simulink model "Teste"  (R2020b)
settings: Solver=VariableStepAuto  StartTime=0.0  StopTime=10.0  RelTol=1e-3
undefined symbols (not defined in the file or in its folder): des, SELECT, T
libraries: simulink x8
(part 3 of 3)

== system Teste/Router5/Clocked FIFO1 ==
  Event-Based Random Number : EventBasedRandomNumber  Distribution=Gaussian (normal)  meanNorm=E  stdNorm=S
  FIFO Queue : FIFOQueue  Capacity=F  StatNumberInBlock=on
      settings: OutputPortMap=o1
  Release Gate : ReleaseGate  OpenGateUpon=Function call from port fcn
  Time-Based Function-Call Generator : TimeBasedFunctionCallGenerator  EventGenerationMode=Period from port  Period=T
  Input : PMIOPort  Side=Left
  Output : PMIOPort  Port=2  Side=Right
  #n : Outport
  wires:
  Event-Based Random Number/1 -> Time-Based Function-Call Generator/1
  FIFO Queue/1 -> #n/1
  Time-Based Function-Call Generator/1 -> Release Gate/1
  connections:
  FIFO Queue/RConn1 -- Release Gate/LConn1
  Release Gate/RConn1 -- Output/RConn1
  FIFO Queue/LConn1 -- Input/RConn1

== system Teste/Router5/Clocked FIFO2 ==
  Event-Based Random Number : EventBasedRandomNumber  Distribution=Gaussian (normal)  meanNorm=E  stdNorm=S
  FIFO Queue : FIFOQueue  Capacity=F  StatNumberInBlock=on
      settings: OutputPortMap=o1
  Release Gate : ReleaseGate  OpenGateUpon=Function call from port fcn
  Time-Based Function-Call Generator : TimeBasedFunctionCallGenerator  EventGenerationMode=Period from port  Period=T
  Input : PMIOPort  Side=Left
  Output : PMIOPort  Port=2  Side=Right
  #n : Outport
  wires:
  Event-Based Random Number/1 -> Time-Based Function-Call Generator/1
  FIFO Queue/1 -> #n/1
  Time-Based Function-Call Generator/1 -> Release Gate/1
  connections:
  FIFO Queue/RConn1 -- Release Gate/LConn1
  Release Gate/RConn1 -- Output/RConn1
  FIFO Queue/LConn1 -- Input/RConn1

== system Teste/Router5/Clocked FIFO3 ==
  Event-Based Random Number : EventBasedRandomNumber  Distribution=Gaussian (normal)  meanNorm=E  stdNorm=S
  FIFO Queue : FIFOQueue  Capacity=F  StatNumberInBlock=on
      settings: OutputPortMap=o1
  Release Gate : ReleaseGate  OpenGateUpon=Function call from port fcn
  Time-Based Function-Call Generator : TimeBasedFunctionCallGenerator  EventGenerationMode=Period from port  Period=T
  Input : PMIOPort  Side=Left
  Output : PMIOPort  Port=2  Side=Right
  #n : Outport
  wires:
  Event-Based Random Number/1 -> Time-Based Function-Call Generator/1
  FIFO Queue/1 -> #n/1
  Time-Based Function-Call Generator/1 -> Release Gate/1
  connections:
  FIFO Queue/RConn1 -- Release Gate/LConn1
  Release Gate/RConn1 -- Output/RConn1
  FIFO Queue/LConn1 -- Input/RConn1

== system Teste/Router5/Clocked FIFO4 ==
  Event-Based Random Number : EventBasedRandomNumber  Distribution=Gaussian (normal)  meanNorm=E  stdNorm=S
  FIFO Queue : FIFOQueue  Capacity=F  StatNumberInBlock=on
      settings: OutputPortMap=o1
  Release Gate : ReleaseGate  OpenGateUpon=Function call from port fcn
  Time-Based Function-Call Generator : TimeBasedFunctionCallGenerator  EventGenerationMode=Period from port  Period=T
  Input : PMIOPort  Side=Left
  Output : PMIOPort  Port=2  Side=Right
  #n : Outport
  wires:
  Event-Based Random Number/1 -> Time-Based Function-Call Generator/1
  FIFO Queue/1 -> #n/1
  Time-Based Function-Call Generator/1 -> Release Gate/1
  connections:
  FIFO Queue/RConn1 -- Release Gate/LConn1
  Release Gate/RConn1 -- Output/RConn1
  FIFO Queue/LConn1 -- Input/RConn1

== system Teste/Router5/Clocked FIFO5 ==
  Event-Based Random Number : EventBasedRandomNumber  Distribution=Gaussian (normal)  meanNorm=E  stdNorm=S
  FIFO Queue : FIFOQueue  Capacity=F  StatNumberInBlock=on
      settings: OutputPortMap=o1
  Release Gate : ReleaseGate  OpenGateUpon=Function call from port fcn
  Time-Based Function-Call Generator : TimeBasedFunctionCallGenerator  EventGenerationMode=Period from port  Period=T
  Input : PMIOPort  Side=Left
  Output : PMIOPort  Port=2  Side=Right
  #n : Outport
  wires:
  Event-Based Random Number/1 -> Time-Based Function-Call Generator/1
  FIFO Queue/1 -> #n/1
  Time-Based Function-Call Generator/1 -> Release Gate/1
  connections:
  FIFO Queue/RConn1 -- Release Gate/LConn1
  Release Gate/RConn1 -- Output/RConn1
  FIFO Queue/LConn1 -- Input/RConn1

== system Teste/Router6/Attribute Function ==
  MATLAB Function : MATLAB Function  TreatAsAtomicUnit=on
  __DMLF__EDE2FCE__ : EntityDepartureFunctionCallGenerator  TimingFunctionCallF1=Before entity departure  IsInsideAFB=on
  __DMLF__GA__ : GetAttribute  AttributeName=DST|ME  AttributeMissing=Error|Error  AttributeDefaultValue=1|1  AttributeTreatAsVector=1|1  AttributeSendTiming=Before entity departure|Before entity departure  EvaluatedDefaultAttributeValue={ [];[]}  IsInsideAFB=on
      settings: OutputPortMap=o1,o2
  __DMLF__SA__ : SetAttribute  AttributeName=RT  AttributeFrom=Signal port  EvaluatedAttributeValue={ []}  IsInsideAFB=on
  IN : PMIOPort  Side=Left
  OUT : PMIOPort  Port=2  Side=Right
  wires:
  MATLAB Function/1(out_RT) -> __DMLF__SA__/1
  __DMLF__GA__/2 -> MATLAB Function/2(ME)
  __DMLF__GA__/1 -> MATLAB Function/1(DST)
  __DMLF__EDE2FCE__/1 -> MATLAB Function/Trigger
  connections:
  __DMLF__SA__/RConn1 -- OUT/RConn1
  IN/RConn1 -- __DMLF__GA__/LConn1
  __DMLF__GA__/RConn1 -- __DMLF__EDE2FCE__/LConn1
  __DMLF__SA__/LConn1 -- __DMLF__EDE2FCE__/RConn1

== system Teste/Router6/Clocked FIFO1 ==
  Event-Based Random Number : EventBasedRandomNumber  Distribution=Gaussian (normal)  meanNorm=E  stdNorm=S
  FIFO Queue : FIFOQueue  Capacity=F  StatNumberInBlock=on
      settings: OutputPortMap=o1
  Release Gate : ReleaseGate  OpenGateUpon=Function call from port fcn
  Time-Based Function-Call Generator : TimeBasedFunctionCallGenerator  EventGenerationMode=Period from port  Period=T
  Input : PMIOPort  Side=Left
  Output : PMIOPort  Port=2  Side=Right
  #n : Outport
  wires:
  Event-Based Random Number/1 -> Time-Based Function-Call Generator/1
  FIFO Queue/1 -> #n/1
  Time-Based Function-Call Generator/1 -> Release Gate/1
  connections:
  FIFO Queue/RConn1 -- Release Gate/LConn1
  Release Gate/RConn1 -- Output/RConn1
  FIFO Queue/LConn1 -- Input/RConn1

== system Teste/Router6/Clocked FIFO2 ==
  Event-Based Random Number : EventBasedRandomNumber  Distribution=Gaussian (normal)  meanNorm=E  stdNorm=S
  FIFO Queue : FIFOQueue  Capacity=F  StatNumberInBlock=on
      settings: OutputPortMap=o1
  Release Gate : ReleaseGate  OpenGateUpon=Function call from port fcn
  Time-Based Function-Call Generator : TimeBasedFunctionCallGenerator  EventGenerationMode=Period from port  Period=T
  Input : PMIOPort  Side=Left
  Output : PMIOPort  Port=2  Side=Right
  #n : Outport
  wires:
  Event-Based Random Number/1 -> Time-Based Function-Call Generator/1
  FIFO Queue/1 -> #n/1
  Time-Based Function-Call Generator/1 -> Release Gate/1
  connections:
  FIFO Queue/RConn1 -- Release Gate/LConn1
  Release Gate/RConn1 -- Output/RConn1
  FIFO Queue/LConn1 -- Input/RConn1

== system Teste/Router6/Clocked FIFO3 ==
  Event-Based Random Number : EventBasedRandomNumber  Distribution=Gaussian (normal)  meanNorm=E  stdNorm=S
  FIFO Queue : FIFOQueue  Capacity=F  StatNumberInBlock=on
      settings: OutputPortMap=o1
  Release Gate : ReleaseGate  OpenGateUpon=Function call from port fcn
  Time-Based Function-Call Generator : TimeBasedFunctionCallGenerator  EventGenerationMode=Period from port  Period=T
  Input : PMIOPort  Side=Left
  Output : PMIOPort  Port=2  Side=Right
  #n : Outport
  wires:
  Event-Based Random Number/1 -> Time-Based Function-Call Generator/1
  FIFO Queue/1 -> #n/1
  Time-Based Function-Call Generator/1 -> Release Gate/1
  connections:
  FIFO Queue/RConn1 -- Release Gate/LConn1
  Release Gate/RConn1 -- Output/RConn1
  FIFO Queue/LConn1 -- Input/RConn1

== system Teste/Router6/Clocked FIFO4 ==
  Event-Based Random Number : EventBasedRandomNumber  Distribution=Gaussian (normal)  meanNorm=E  stdNorm=S
  FIFO Queue : FIFOQueue  Capacity=F  StatNumberInBlock=on
      settings: OutputPortMap=o1
  Release Gate : ReleaseGate  OpenGateUpon=Function call from port fcn
  Time-Based Function-Call Generator : TimeBasedFunctionCallGenerator  EventGenerationMode=Period from port  Period=T
  Input : PMIOPort  Side=Left
  Output : PMIOPort  Port=2  Side=Right
  #n : Outport
  wires:
  Event-Based Random Number/1 -> Time-Based Function-Call Generator/1
  FIFO Queue/1 -> #n/1
  Time-Based Function-Call Generator/1 -> Release Gate/1
  connections:
  FIFO Queue/RConn1 -- Release Gate/LConn1
  Release Gate/RConn1 -- Output/RConn1
  FIFO Queue/LConn1 -- Input/RConn1

== system Teste/Router6/Clocked FIFO5 ==
  Event-Based Random Number : EventBasedRandomNumber  Distribution=Gaussian (normal)  meanNorm=E  stdNorm=S
  FIFO Queue : FIFOQueue  Capacity=F  StatNumberInBlock=on
      settings: OutputPortMap=o1
  Release Gate : ReleaseGate  OpenGateUpon=Function call from port fcn
  Time-Based Function-Call Generator : TimeBasedFunctionCallGenerator  EventGenerationMode=Period from port  Period=T
  Input : PMIOPort  Side=Left
  Output : PMIOPort  Port=2  Side=Right
  #n : Outport
  wires:
  Event-Based Random Number/1 -> Time-Based Function-Call Generator/1
  FIFO Queue/1 -> #n/1
  Time-Based Function-Call Generator/1 -> Release Gate/1
  connections:
  FIFO Queue/RConn1 -- Release Gate/LConn1
  Release Gate/RConn1 -- Output/RConn1
  FIFO Queue/LConn1 -- Input/RConn1

== system Teste/Router7/Attribute Function ==
  MATLAB Function : MATLAB Function  TreatAsAtomicUnit=on
  __DMLF__EDE2FCE__ : EntityDepartureFunctionCallGenerator  TimingFunctionCallF1=Before entity departure  IsInsideAFB=on
  __DMLF__GA__ : GetAttribute  AttributeName=DST|ME  AttributeMissing=Error|Error  AttributeDefaultValue=1|1  AttributeTreatAsVector=1|1  AttributeSendTiming=Before entity departure|Before entity departure  EvaluatedDefaultAttributeValue={ [];[]}  IsInsideAFB=on
      settings: OutputPortMap=o1,o2
  __DMLF__SA__ : SetAttribute  AttributeName=RT  AttributeFrom=Signal port  EvaluatedAttributeValue={ []}  IsInsideAFB=on
  IN : PMIOPort  Side=Left
  OUT : PMIOPort  Port=2  Side=Right
  wires:
  MATLAB Function/1(out_RT) -> __DMLF__SA__/1
  __DMLF__GA__/2 -> MATLAB Function/2(ME)
  __DMLF__GA__/1 -> MATLAB Function/1(DST)
  __DMLF__EDE2FCE__/1 -> MATLAB Function/Trigger
  connections:
  __DMLF__SA__/RConn1 -- OUT/RConn1
  IN/RConn1 -- __DMLF__GA__/LConn1
  __DMLF__GA__/RConn1 -- __DMLF__EDE2FCE__/LConn1
  __DMLF__SA__/LConn1 -- __DMLF__EDE2FCE__/RConn1

== system Teste/Router7/Clocked FIFO1 ==
  Event-Based Random Number : EventBasedRandomNumber  Distribution=Gaussian (normal)  meanNorm=E  stdNorm=S
  FIFO Queue : FIFOQueue  Capacity=F  StatNumberInBlock=on
      settings: OutputPortMap=o1
  Release Gate : ReleaseGate  OpenGateUpon=Function call from port fcn
  Time-Based Function-Call Generator : TimeBasedFunctionCallGenerator  EventGenerationMode=Period from port  Period=T
  Input : PMIOPort  Side=Left
  Output : PMIOPort  Port=2  Side=Right
  #n : Outport
  wires:
  Event-Based Random Number/1 -> Time-Based Function-Call Generator/1
  FIFO Queue/1 -> #n/1
  Time-Based Function-Call Generator/1 -> Release Gate/1
  connections:
  FIFO Queue/RConn1 -- Release Gate/LConn1
  Release Gate/RConn1 -- Output/RConn1
  FIFO Queue/LConn1 -- Input/RConn1

== system Teste/Router7/Clocked FIFO2 ==
  Event-Based Random Number : EventBasedRandomNumber  Distribution=Gaussian (normal)  meanNorm=E  stdNorm=S
  FIFO Queue : FIFOQueue  Capacity=F  StatNumberInBlock=on
      settings: OutputPortMap=o1
  Release Gate : ReleaseGate  OpenGateUpon=Function call from port fcn
  Time-Based Function-Call Generator : TimeBasedFunctionCallGenerator  EventGenerationMode=Period from port  Period=T
  Input : PMIOPort  Side=Left
  Output : PMIOPort  Port=2  Side=Right
  #n : Outport
  wires:
  Event-Based Random Number/1 -> Time-Based Function-Call Generator/1
  FIFO Queue/1 -> #n/1
  Time-Based Function-Call Generator/1 -> Release Gate/1
  connections:
  FIFO Queue/RConn1 -- Release Gate/LConn1
  Release Gate/RConn1 -- Output/RConn1
  FIFO Queue/LConn1 -- Input/RConn1

== system Teste/Router7/Clocked FIFO3 ==
  Event-Based Random Number : EventBasedRandomNumber  Distribution=Gaussian (normal)  meanNorm=E  stdNorm=S
  FIFO Queue : FIFOQueue  Capacity=F  StatNumberInBlock=on
      settings: OutputPortMap=o1
  Release Gate : ReleaseGate  OpenGateUpon=Function call from port fcn
  Time-Based Function-Call Generator : TimeBasedFunctionCallGenerator  EventGenerationMode=Period from port  Period=T
  Input : PMIOPort  Side=Left
  Output : PMIOPort  Port=2  Side=Right
  #n : Outport
  wires:
  Event-Based Random Number/1 -> Time-Based Function-Call Generator/1
  FIFO Queue/1 -> #n/1
  Time-Based Function-Call Generator/1 -> Release Gate/1
  connections:
  FIFO Queue/RConn1 -- Release Gate/LConn1
  Release Gate/RConn1 -- Output/RConn1
  FIFO Queue/LConn1 -- Input/RConn1

== system Teste/Router7/Clocked FIFO4 ==
  Event-Based Random Number : EventBasedRandomNumber  Distribution=Gaussian (normal)  meanNorm=E  stdNorm=S
  FIFO Queue : FIFOQueue  Capacity=F  StatNumberInBlock=on
      settings: OutputPortMap=o1
  Release Gate : ReleaseGate  OpenGateUpon=Function call from port fcn
  Time-Based Function-Call Generator : TimeBasedFunctionCallGenerator  EventGenerationMode=Period from port  Period=T
  Input : PMIOPort  Side=Left
  Output : PMIOPort  Port=2  Side=Right
  #n : Outport
  wires:
  Event-Based Random Number/1 -> Time-Based Function-Call Generator/1
  FIFO Queue/1 -> #n/1
  Time-Based Function-Call Generator/1 -> Release Gate/1
  connections:
  FIFO Queue/RConn1 -- Release Gate/LConn1
  Release Gate/RConn1 -- Output/RConn1
  FIFO Queue/LConn1 -- Input/RConn1

== system Teste/Router7/Clocked FIFO5 ==
  Event-Based Random Number : EventBasedRandomNumber  Distribution=Gaussian (normal)  meanNorm=E  stdNorm=S
  FIFO Queue : FIFOQueue  Capacity=F  StatNumberInBlock=on
      settings: OutputPortMap=o1
  Release Gate : ReleaseGate  OpenGateUpon=Function call from port fcn
  Time-Based Function-Call Generator : TimeBasedFunctionCallGenerator  EventGenerationMode=Period from port  Period=T
  Input : PMIOPort  Side=Left
  Output : PMIOPort  Port=2  Side=Right
  #n : Outport
  wires:
  Event-Based Random Number/1 -> Time-Based Function-Call Generator/1
  FIFO Queue/1 -> #n/1
  Time-Based Function-Call Generator/1 -> Release Gate/1
  connections:
  FIFO Queue/RConn1 -- Release Gate/LConn1
  Release Gate/RConn1 -- Output/RConn1
  FIFO Queue/LConn1 -- Input/RConn1

== system Teste/Router8/Attribute Function ==
  MATLAB Function : MATLAB Function  TreatAsAtomicUnit=on
  __DMLF__EDE2FCE__ : EntityDepartureFunctionCallGenerator  TimingFunctionCallF1=Before entity departure  IsInsideAFB=on
  __DMLF__GA__ : GetAttribute  AttributeName=DST|ME  AttributeMissing=Error|Error  AttributeDefaultValue=1|1  AttributeTreatAsVector=1|1  AttributeSendTiming=Before entity departure|Before entity departure  EvaluatedDefaultAttributeValue={ [];[]}  IsInsideAFB=on
      settings: OutputPortMap=o1,o2
  __DMLF__SA__ : SetAttribute  AttributeName=RT  AttributeFrom=Signal port  EvaluatedAttributeValue={ []}  IsInsideAFB=on
  IN : PMIOPort  Side=Left
  OUT : PMIOPort  Port=2  Side=Right
  wires:
  MATLAB Function/1(out_RT) -> __DMLF__SA__/1
  __DMLF__GA__/2 -> MATLAB Function/2(ME)
  __DMLF__GA__/1 -> MATLAB Function/1(DST)
  __DMLF__EDE2FCE__/1 -> MATLAB Function/Trigger
  connections:
  __DMLF__SA__/RConn1 -- OUT/RConn1
  IN/RConn1 -- __DMLF__GA__/LConn1
  __DMLF__GA__/RConn1 -- __DMLF__EDE2FCE__/LConn1
  __DMLF__SA__/LConn1 -- __DMLF__EDE2FCE__/RConn1

== system Teste/Router8/Clocked FIFO1 ==
  Event-Based Random Number : EventBasedRandomNumber  Distribution=Gaussian (normal)  meanNorm=E  stdNorm=S
  FIFO Queue : FIFOQueue  Capacity=F  StatNumberInBlock=on
      settings: OutputPortMap=o1
  Release Gate : ReleaseGate  OpenGateUpon=Function call from port fcn
  Time-Based Function-Call Generator : TimeBasedFunctionCallGenerator  EventGenerationMode=Period from port  Period=T
  Input : PMIOPort  Side=Left
  Output : PMIOPort  Port=2  Side=Right
  #n : Outport
  wires:
  Event-Based Random Number/1 -> Time-Based Function-Call Generator/1
  FIFO Queue/1 -> #n/1
  Time-Based Function-Call Generator/1 -> Release Gate/1
  connections:
  FIFO Queue/RConn1 -- Release Gate/LConn1
  Release Gate/RConn1 -- Output/RConn1
  FIFO Queue/LConn1 -- Input/RConn1

== system Teste/Router8/Clocked FIFO2 ==
  Event-Based Random Number : EventBasedRandomNumber  Distribution=Gaussian (normal)  meanNorm=E  stdNorm=S
  FIFO Queue : FIFOQueue  Capacity=F  StatNumberInBlock=on
      settings: OutputPortMap=o1
  Release Gate : ReleaseGate  OpenGateUpon=Function call from port fcn
  Time-Based Function-Call Generator : TimeBasedFunctionCallGenerator  EventGenerationMode=Period from port  Period=T
  Input : PMIOPort  Side=Left
  Output : PMIOPort  Port=2  Side=Right
  #n : Outport
  wires:
  Event-Based Random Number/1 -> Time-Based Function-Call Generator/1
  FIFO Queue/1 -> #n/1
  Time-Based Function-Call Generator/1 -> Release Gate/1
  connections:
  FIFO Queue/RConn1 -- Release Gate/LConn1
  Release Gate/RConn1 -- Output/RConn1
  FIFO Queue/LConn1 -- Input/RConn1

== system Teste/Router8/Clocked FIFO3 ==
  Event-Based Random Number : EventBasedRandomNumber  Distribution=Gaussian (normal)  meanNorm=E  stdNorm=S
  FIFO Queue : FIFOQueue  Capacity=F  StatNumberInBlock=on
      settings: OutputPortMap=o1
  Release Gate : ReleaseGate  OpenGateUpon=Function call from port fcn
  Time-Based Function-Call Generator : TimeBasedFunctionCallGenerator  EventGenerationMode=Period from port  Period=T
  Input : PMIOPort  Side=Left
  Output : PMIOPort  Port=2  Side=Right
  #n : Outport
  wires:
  Event-Based Random Number/1 -> Time-Based Function-Call Generator/1
  FIFO Queue/1 -> #n/1
  Time-Based Function-Call Generator/1 -> Release Gate/1
  connections:
  FIFO Queue/RConn1 -- Release Gate/LConn1
  Release Gate/RConn1 -- Output/RConn1
  FIFO Queue/LConn1 -- Input/RConn1

== system Teste/Router8/Clocked FIFO4 ==
  Event-Based Random Number : EventBasedRandomNumber  Distribution=Gaussian (normal)  meanNorm=E  stdNorm=S
  FIFO Queue : FIFOQueue  Capacity=F  StatNumberInBlock=on
      settings: OutputPortMap=o1
  Release Gate : ReleaseGate  OpenGateUpon=Function call from port fcn
  Time-Based Function-Call Generator : TimeBasedFunctionCallGenerator  EventGenerationMode=Period from port  Period=T
  Input : PMIOPort  Side=Left
  Output : PMIOPort  Port=2  Side=Right
  #n : Outport
  wires:
  Event-Based Random Number/1 -> Time-Based Function-Call Generator/1
  FIFO Queue/1 -> #n/1
  Time-Based Function-Call Generator/1 -> Release Gate/1
  connections:
  FIFO Queue/RConn1 -- Release Gate/LConn1
  Release Gate/RConn1 -- Output/RConn1
  FIFO Queue/LConn1 -- Input/RConn1

== system Teste/Router8/Clocked FIFO5 ==
  Event-Based Random Number : EventBasedRandomNumber  Distribution=Gaussian (normal)  meanNorm=E  stdNorm=S
  FIFO Queue : FIFOQueue  Capacity=F  StatNumberInBlock=on
      settings: OutputPortMap=o1
  Release Gate : ReleaseGate  OpenGateUpon=Function call from port fcn
  Time-Based Function-Call Generator : TimeBasedFunctionCallGenerator  EventGenerationMode=Period from port  Period=T
  Input : PMIOPort  Side=Left
  Output : PMIOPort  Port=2  Side=Right
  #n : Outport
  wires:
  Event-Based Random Number/1 -> Time-Based Function-Call Generator/1
  FIFO Queue/1 -> #n/1
  Time-Based Function-Call Generator/1 -> Release Gate/1
  connections:
  FIFO Queue/RConn1 -- Release Gate/LConn1
  Release Gate/RConn1 -- Output/RConn1
  FIFO Queue/LConn1 -- Input/RConn1

== matlab function Teste/Router1/Attribute Function/MATLAB Function ==
  data: DST input; out_RT output; ME input
  events: trigger input FUNCTION_CALL_EVENT
function out_RT  = fcn(DST,ME)
%FCN    Access and modify attributes with MATLAB 
% 
% Input arguments must match the attribute names.
% Output arguments must be out_<AttributeName>,
% e.g., out_ServiceTime where ServiceTime is the attribute name.
% 
% The output attribute will be created if it is not present.
%

yi = floor(ME/4)+1;
xi = mod(ME,4);

if (xi==0),
    xi = 4;
    yi = yi - 1;
end

y = floor(DST/4)+1;
x = mod(DST,4);

if (x==0),
   x = 4;
    y = y - 1;
end

if x~=xi,
    if (x<xi),
        out_RT = 2;
    else 
        out_RT = 3;
    end
elseif y~=yi,
    if (y<yi),
        out_RT = 1;
    else
        out_RT = 4;
    end
else
    out_RT = 5;
end

== matlab function Teste/Router2/Attribute Function/MATLAB Function ==
  data: DST input; out_RT output; ME input
  events: trigger input FUNCTION_CALL_EVENT
function out_RT  = fcn(DST,ME)
%FCN    Access and modify attributes with MATLAB 
% 
% Input arguments must match the attribute names.
% Output arguments must be out_<AttributeName>,
% e.g., out_ServiceTime where ServiceTime is the attribute name.
% 
% The output attribute will be created if it is not present.
%

yi = floor(ME/4)+1;
xi = mod(ME,4);

if (xi==0),
    xi = 4;
    yi = yi - 1;
end

y = floor(DST/4)+1;
x = mod(DST,4);

if (x==0),
   x = 4;
    y = y - 1;
end

if x~=xi,
    if (x<xi),
        out_RT = 2;
    else 
        out_RT = 3;
    end
elseif y~=yi,
    if (y<yi),
        out_RT = 1;
    else
        out_RT = 4;
    end
else
    out_RT = 5;
end

== matlab function Teste/Router3/Attribute Function/MATLAB Function ==
  data: DST input; out_RT output; ME input
  events: trigger input FUNCTION_CALL_EVENT
function out_RT  = fcn(DST,ME)
%FCN    Access and modify attributes with MATLAB 
% 
% Input arguments must match the attribute names.
% Output arguments must be out_<AttributeName>,
% e.g., out_ServiceTime where ServiceTime is the attribute name.
% 
% The output attribute will be created if it is not present.
%

yi = floor(ME/4)+1;
xi = mod(ME,4);

if (xi==0),
    xi = 4;
    yi = yi - 1;
end

y = floor(DST/4)+1;
x = mod(DST,4);

if (x==0),
   x = 4;
    y = y - 1;
end

if x~=xi,
    if (x<xi),
        out_RT = 2;
    else 
        out_RT = 3;
    end
elseif y~=yi,
    if (y<yi),
        out_RT = 1;
    else
        out_RT = 4;
    end
else
    out_RT = 5;
end

== matlab function Teste/Router4/Attribute Function/MATLAB Function ==
  data: DST input; out_RT output; ME input
  events: trigger input FUNCTION_CALL_EVENT
function out_RT  = fcn(DST,ME)
%FCN    Access and modify attributes with MATLAB 
% 
% Input arguments must match the attribute names.
% Output arguments must be out_<AttributeName>,
% e.g., out_ServiceTime where ServiceTime is the attribute name.
% 
% The output attribute will be created if it is not present.
%

yi = floor(ME/4)+1;
xi = mod(ME,4);

if (xi==0),
    xi = 4;
    yi = yi - 1;
end

y = floor(DST/4)+1;
x = mod(DST,4);

if (x==0),
   x = 4;
    y = y - 1;
end

if x~=xi,
    if (x<xi),
        out_RT = 2;
    else 
        out_RT = 3;
    end
elseif y~=yi,
    if (y<yi),
        out_RT = 1;
    else
        out_RT = 4;
    end
else
    out_RT = 5;
end

== matlab function Teste/Router5/Attribute Function/MATLAB Function ==
  data: DST input; out_RT output; ME input
  events: trigger input FUNCTION_CALL_EVENT
function out_RT  = fcn(DST,ME)
%FCN    Access and modify attributes with MATLAB 
% 
% Input arguments must match the attribute names.
% Output arguments must be out_<AttributeName>,
% e.g., out_ServiceTime where ServiceTime is the attribute name.
% 
% The output attribute will be created if it is not present.
%

yi = floor(ME/4)+1;
xi = mod(ME,4);

if (xi==0),
    xi = 4;
    yi = yi - 1;
end

y = floor(DST/4)+1;
x = mod(DST,4);

if (x==0),
   x = 4;
    y = y - 1;
end

if x~=xi,
    if (x<xi),
        out_RT = 2;
    else 
        out_RT = 3;
    end
elseif y~=yi,
    if (y<yi),
        out_RT = 1;
    else
        out_RT = 4;
    end
else
    out_RT = 5;
end

== matlab function Teste/Router6/Attribute Function/MATLAB Function ==
  data: DST input; out_RT output; ME input
  events: trigger input FUNCTION_CALL_EVENT
function out_RT  = fcn(DST,ME)
%FCN    Access and modify attributes with MATLAB 
% 
% Input arguments must match the attribute names.
% Output arguments must be out_<AttributeName>,
% e.g., out_ServiceTime where ServiceTime is the attribute name.
% 
% The output attribute will be created if it is not present.
%

yi = floor(ME/4)+1;
xi = mod(ME,4);

if (xi==0),
    xi = 4;
    yi = yi - 1;
end

y = floor(DST/4)+1;
x = mod(DST,4);

if (x==0),
   x = 4;
    y = y - 1;
end

if x~=xi,
    if (x<xi),
        out_RT = 2;
    else 
        out_RT = 3;
    end
elseif y~=yi,
    if (y<yi),
        out_RT = 1;
    else
        out_RT = 4;
    end
else
    out_RT = 5;
end

== matlab function Teste/Router7/Attribute Function/MATLAB Function ==
  data: DST input; out_RT output; ME input
  events: trigger input FUNCTION_CALL_EVENT
function out_RT  = fcn(DST,ME)
%FCN    Access and modify attributes with MATLAB 
% 
% Input arguments must match the attribute names.
% Output arguments must be out_<AttributeName>,
% e.g., out_ServiceTime where ServiceTime is the attribute name.
% 
% The output attribute will be created if it is not present.
%

yi = floor(ME/4)+1;
xi = mod(ME,4);

if (xi==0),
    xi = 4;
    yi = yi - 1;
end

y = floor(DST/4)+1;
x = mod(DST,4);

if (x==0),
   x = 4;
    y = y - 1;
end

if x~=xi,
    if (x<xi),
        out_RT = 2;
    else 
        out_RT = 3;
    end
elseif y~=yi,
    if (y<yi),
        out_RT = 1;
    else
        out_RT = 4;
    end
else
    out_RT = 5;
end

== matlab function Teste/Router8/Attribute Function/MATLAB Function ==
  data: DST input; out_RT output; ME input
  events: trigger input FUNCTION_CALL_EVENT
function out_RT  = fcn(DST,ME)
%FCN    Access and modify attributes with MATLAB 
% 
% Input arguments must match the attribute names.
% Output arguments must be out_<AttributeName>,
% e.g., out_ServiceTime where ServiceTime is the attribute name.
% 
% The output attribute will be created if it is not present.
%

yi = floor(ME/4)+1;
xi = mod(ME,4);

if (xi==0),
    xi = 4;
    yi = yi - 1;
end

y = floor(DST/4)+1;
x = mod(DST,4);

if (x==0),
   x = 4;
    y = y - 1;
end

if x~=xi,
    if (x<xi),
        out_RT = 2;
    else 
        out_RT = 3;
    end
elseif y~=yi,
    if (y<yi),
        out_RT = 1;
    else
        out_RT = 4;
    end
else
    out_RT = 5;
end
